simulink model "RMU22"  (R2025b)
settings: Solver=VariableStepAuto  StartTime=0.0  StopTime=12  RelTol=1e-3
libraries: spsThreePhaseBreakerLib x11, spsThreePhaseParallelRLCLoadLib x6, spsThreePhasePISectionLineLib x6, spsThreePhaseFaultLib x3, spsThreePhaseVIMeasurementLib x3, spsThreePhaseSourceLib x2, spsThreePhaseTransformerTwoWindingsLib x2, sps_lib x1
settings Model: Creator=sheya  LastModifiedBy=josna_mz

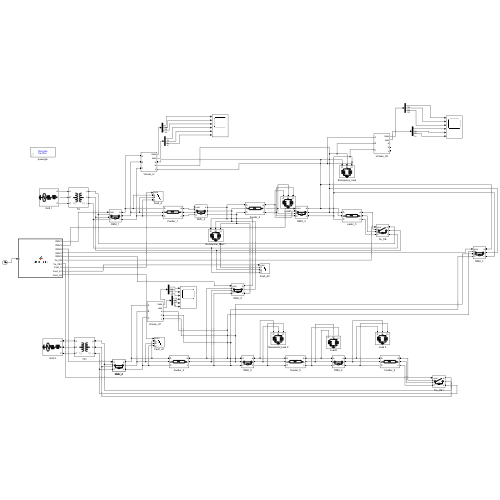
[thumbnail: Simulink's stored preview of the top-level diagram]
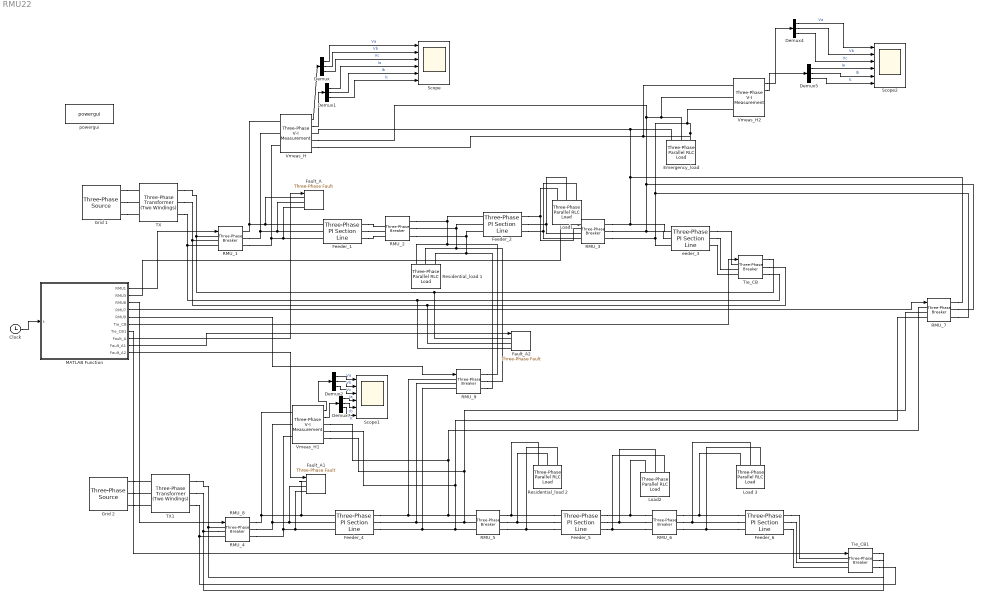
== system RMU22 ==
  Clock : Clock
  Demux{,1..5} (6 alike) : Demux  Outputs=3
  Emergency_load : spsThreePhaseParallelRLCLoadLib/Three-Phase Parallel RLC Load  LConnTagsString=A|B|C  Configuration=Y (grounded)  NominalVoltage=11000  Vabc=[1e3 1e3 1e3]  Vabcp=[1e3 1e3 1e3]  NominalFrequency=60  UnbalancedPower=off  ActivePower=5e5  InductivePower=1.64e5  CapacitivePower=0  Pabc=[10e3 9e3 11e3]  QLabc=[100 90 110]  QCabc=[100 90 110]  Pabcp=[10e3 9e3 11e3]  QLabcp=[100 90 110]  QCabcp=[100 90 110]  Measurements=None  LoadType=constant Z
  Fault_A : spsThreePhaseFaultLib/Three-Phase Fault  InitialStates=0  FaultA=on  FaultB=on  FaultC=on  GroundFault=on  SwitchTimes="[0.2  0.5]"  External=on  SwitchStatus=NaN  FaultResistance=0.001  GroundResistance=0.01  SnubberResistance=1e6  SnubberCapacitance=inf  Measurements=None
  Fault_A1 : spsThreePhaseFaultLib/Three-Phase Fault  InitialStates=0  FaultA=on  FaultB=on  FaultC=on  GroundFault=on  SwitchTimes="[0.2  0.5]"  External=on  SwitchStatus=NaN  FaultResistance=0.001  GroundResistance=0.01  SnubberResistance=1e6  SnubberCapacitance=inf  Measurements=None
  Fault_A2 : spsThreePhaseFaultLib/Three-Phase Fault  InitialStates=0  FaultA=on  FaultB=on  FaultC=on  GroundFault=on  SwitchTimes="[0.2  0.5]"  External=on  SwitchStatus=NaN  FaultResistance=0.001  GroundResistance=0.01  SnubberResistance=1e6  SnubberCapacitance=inf  Measurements=None
  Feeder_{1..2,4..6} (5 alike) : spsThreePhasePISectionLineLib/Three-Phase PI Section Line  LConnTagsString=a|b|c  RConnTagsString=A|B|C  Length=100  Frequency=60  Resistances=[ 0.01273 0.3864]  Inductances="[ 0.9337e-3  4.1264e-3]"  Capacitances=[12.74e-9 7.751e-9]
  Grid 1 : spsThreePhaseSourceLib/Three-Phase Source  InternalConnection=Yg  VoltagePhases=off  Voltage=11000  PhaseAngle=0  Voltage_phases=[25e3 25e3 25e3]/sqrt(3)  PhaseAngles_phases=[0 -120 +120]  Frequency=50  NonIdealSource=on  SpecifyImpedance=off  Resistance=0.8929  Inductance=16.58e-3  ShortCircuitLevel=100e6  BaseVoltage=25e3  XRratio=7  BusType=swing  Pref=10e3  Qref=0  Prefabc=[10e3, 10e3, 10e3]  Qrefabc=[0, 0, 0]  Qmin=-inf  Qmax=inf
  Grid 2 : spsThreePhaseSourceLib/Three-Phase Source  InternalConnection=Yg  VoltagePhases=off  Voltage=11000  PhaseAngle=0  Voltage_phases=[25e3 25e3 25e3]/sqrt(3)  PhaseAngles_phases=[0 -120 +120]  Frequency=50  NonIdealSource=on  SpecifyImpedance=off  Resistance=0.8929  Inductance=16.58e-3  ShortCircuitLevel=100e6  BaseVoltage=25e3  XRratio=7  BusType=swing  Pref=10e3  Qref=0  Prefabc=[10e3, 10e3, 10e3]  Qrefabc=[0, 0, 0]  Qmin=-inf  Qmax=inf
  Load 3 : spsThreePhaseParallelRLCLoadLib/Three-Phase Parallel RLC Load  LConnTagsString=A|B|C  Configuration=Y (grounded)  NominalVoltage=11000  Vabc=[1e3 1e3 1e3]  Vabcp=[1e3 1e3 1e3]  NominalFrequency=60  UnbalancedPower=off  ActivePower=7e5  InductivePower=3.77e5  CapacitivePower=0  Pabc=[10e3 9e3 11e3]  QLabc=[100 90 110]  QCabc=[100 90 110]  Pabcp=[10e3 9e3 11e3]  QLabcp=[100 90 110]  QCabcp=[100 90 110]  Measurements=None  LoadType=constant Z
  Load1 : spsThreePhaseParallelRLCLoadLib/Three-Phase Parallel RLC Load  LConnTagsString=A|B|C  Configuration=Y (grounded)  NominalVoltage=11000  Vabc=[1e3 1e3 1e3]  Vabcp=[1e3 1e3 1e3]  NominalFrequency=60  UnbalancedPower=off  ActivePower=6e5  InductivePower=3.71e5  CapacitivePower=0  Pabc=[10e3 9e3 11e3]  QLabc=[100 90 110]  QCabc=[100 90 110]  Pabcp=[10e3 9e3 11e3]  QLabcp=[100 90 110]  QCabcp=[100 90 110]  Measurements=None  LoadType=constant Z
  Load2 : spsThreePhaseParallelRLCLoadLib/Three-Phase Parallel RLC Load  LConnTagsString=A|B|C  Configuration=Y (grounded)  NominalVoltage=11000  Vabc=[1e3 1e3 1e3]  Vabcp=[1e3 1e3 1e3]  NominalFrequency=60  UnbalancedPower=off  ActivePower=5e5  InductivePower=2.42e5  CapacitivePower=0  Pabc=[10e3 9e3 11e3]  QLabc=[100 90 110]  QCabc=[100 90 110]  Pabcp=[10e3 9e3 11e3]  QLabcp=[100 90 110]  QCabcp=[100 90 110]  Measurements=None  LoadType=constant Z
  MATLAB Function : MATLAB Function  TreatAsAtomicUnit=on
  RMU_{1..4,7,9} (6 alike) : spsThreePhaseBreakerLib/Three-Phase Breaker  InitialState=closed  SwitchA=on  SwitchB=on  SwitchC=on  SwitchTimes="[1/60  5/60]"  External=on  BreakerResistance=0.01  SnubberResistance=1e6  SnubberCapacitance=inf  Measurements=None
  RMU_5 : spsThreePhaseBreakerLib/Three-Phase Breaker  InitialState=closed  SwitchA=on  SwitchB=on  SwitchC=on  SwitchTimes="[1/60  5/60]"  External=off  BreakerResistance=0.01  SnubberResistance=1e6  SnubberCapacitance=inf  Measurements=None
  RMU_6 : spsThreePhaseBreakerLib/Three-Phase Breaker  InitialState=closed  SwitchA=on  SwitchB=on  SwitchC=on  SwitchTimes="[1/60  5/60]"  External=off  BreakerResistance=0.01  SnubberResistance=1e6  SnubberCapacitance=inf  Measurements=None
  RMU_8 : spsThreePhaseBreakerLib/Three-Phase Breaker  InitialState=closed  SwitchA=on  SwitchB=on  SwitchC=on  SwitchTimes="[1/60  5/60]"  External=off  BreakerResistance=0.01  SnubberResistance=1e6  SnubberCapacitance=inf  Measurements=None
  Residential_load 1 : spsThreePhaseParallelRLCLoadLib/Three-Phase Parallel RLC Load  LConnTagsString=A|B|C  Configuration=Y (grounded)  NominalVoltage=11000  Vabc=[1e3 1e3 1e3]  Vabcp=[1e3 1e3 1e3]  NominalFrequency=60  UnbalancedPower=off  ActivePower=9e5  InductivePower=4.36e5  CapacitivePower=0  Pabc=[10e3 9e3 11e3]  QLabc=[100 90 110]  QCabc=[100 90 110]  Pabcp=[10e3 9e3 11e3]  QLabcp=[100 90 110]  QCabcp=[100 90 110]  Measurements=None  LoadType=constant Z
  Residential_load 2 : spsThreePhaseParallelRLCLoadLib/Three-Phase Parallel RLC Load  LConnTagsString=A|B|C  Configuration=Y (grounded)  NominalVoltage=11000  Vabc=[1e3 1e3 1e3]  Vabcp=[1e3 1e3 1e3]  NominalFrequency=60  UnbalancedPower=off  ActivePower=8e5  InductivePower=3.87e5  CapacitivePower=0  Pabc=[10e3 9e3 11e3]  QLabc=[100 90 110]  QCabc=[100 90 110]  Pabcp=[10e3 9e3 11e3]  QLabcp=[100 90 110]  QCabcp=[100 90 110]  Measurements=None  LoadType=constant Z
  Scope : Scope  NumInputPorts=6
      settings: ActiveDisplayYMinimum=-1  ActiveDisplayYMaximum=1  YLabel=Voltage (Volts)
  Scope1 : Scope  NumInputPorts=6
      settings: ActiveDisplayYMinimum=-6112.8015624898089  ActiveDisplayYMaximum=6194.6590194442269  YLabel=Voltage (Volts)
  Scope2 : Scope  NumInputPorts=6
      settings: ActiveDisplayYMinimum=-1  ActiveDisplayYMaximum=1  YLabel=Voltage (Volts)  DataLoggingVariableName=ScopeData2
  TX : spsThreePhaseTransformerTwoWindingsLib/Three-Phase Transformer (Two Windings)  Winding1Connection=Yg  Winding2Connection=Yg  CoreType=Three single-phase transformers  SetSaturation=off  Hysteresis=off  DataFile='hysteresis'  SetInitialFlux=off  Measurements=None  UNITS=pu  NominalPower=[ 250e6 , 60 ]  Winding1=[ 735e3 , 0.002 , 0.08 ]  Winding2=[ 315e3 , 0.002 , 0.08 ]  Rm=500  Lm=500  L0=0.5  Saturation=[ 0,0 ; 0.0024,1.2 ; 1.0,1.52 ]  InitialFluxes=[ 0.8 , -0.8 , 0.7 ]  BreakLoop=off  DiscreteSolver=Trapezoidal iterative  DataType=off  TransfoNumber=1
  TX1 : spsThreePhaseTransformerTwoWindingsLib/Three-Phase Transformer (Two Windings)  Winding1Connection=Yg  Winding2Connection=Yg  CoreType=Three single-phase transformers  SetSaturation=off  Hysteresis=off  DataFile='hysteresis'  SetInitialFlux=off  Measurements=None  UNITS=pu  NominalPower=[ 250e6 , 60 ]  Winding1=[ 735e3 , 0.002 , 0.08 ]  Winding2=[ 315e3 , 0.002 , 0.08 ]  Rm=500  Lm=500  L0=0.5  Saturation=[ 0,0 ; 0.0024,1.2 ; 1.0,1.52 ]  InitialFluxes=[ 0.8 , -0.8 , 0.7 ]  BreakLoop=off  DiscreteSolver=Trapezoidal iterative  DataType=off  TransfoNumber=1
  Tie_CB : spsThreePhaseBreakerLib/Three-Phase Breaker  InitialState=open  SwitchA=on  SwitchB=on  SwitchC=on  SwitchTimes="[1/60  5/60]"  External=on  BreakerResistance=0.01  SnubberResistance=1e6  SnubberCapacitance=inf  Measurements=None
  Tie_CB1 : spsThreePhaseBreakerLib/Three-Phase Breaker  InitialState=open  SwitchA=on  SwitchB=on  SwitchC=on  SwitchTimes="[1/60  5/60]"  External=on  BreakerResistance=0.01  SnubberResistance=1e6  SnubberCapacitance=inf  Measurements=None
  Vmeas_H : spsThreePhaseVIMeasurementLib/Three-Phase V-I Measurement  VoltageMeasurement=phase-to-ground  SetLabelV=off  LabelV=Vabc  Vpu=off  VpuLL=off  CurrentMeasurement=yes  SetLabelI=off  LabelI=Iabc  Ipu=off  Pbase=100e6  Vbase=500e3  OutputType=Complex  PhasorSimulation=off  PSBequivalent=0
  Vmeas_H1 : spsThreePhaseVIMeasurementLib/Three-Phase V-I Measurement  VoltageMeasurement=phase-to-ground  SetLabelV=off  LabelV=Vabc  Vpu=off  VpuLL=off  CurrentMeasurement=yes  SetLabelI=off  LabelI=Iabc  Ipu=off  Pbase=100e6  Vbase=500e3  OutputType=Complex  PhasorSimulation=off  PSBequivalent=0
  Vmeas_H2 : spsThreePhaseVIMeasurementLib/Three-Phase V-I Measurement  VoltageMeasurement=phase-to-ground  SetLabelV=off  LabelV=Vabc  Vpu=off  VpuLL=off  CurrentMeasurement=yes  SetLabelI=off  LabelI=Iabc  Ipu=off  Pbase=100e6  Vbase=500e3  OutputType=Complex  PhasorSimulation=off  PSBequivalent=0
  eeder_3 : spsThreePhasePISectionLineLib/Three-Phase PI Section Line  LConnTagsString=a|b|c  RConnTagsString=A|B|C  Length=100  Frequency=60  Resistances=[ 0.01273 0.3864]  Inductances="[ 0.9337e-3  4.1264e-3]"  Capacitances=[12.74e-9 7.751e-9]
  powergui : sps_lib/powergui  Priority=1  SimulationMode=Discrete  SampleTime=50e-6  frequency=60  Iterations=50  frequencyindice=0  Pbase=100e6  ErrMax=1e-4  UnitsV=kV  UnitsW=MW  buscounter=0  FunctionMessages=off  echomessages=off  EnableUseOfTLC=off  CurrentSourceSwitches=off  DisableSnubberDevices=off  DisableRonSwitches=off  DisableVfSwitches=off  DisplayEquations=off  AutomaticDiscreteSolvers=off  SolverType=Tustin/Backward Euler (TBE)  Interpol=off  ExternalGateDelay=off  methode=off  Ts=100  x0status=blocks  SPID=on  SwTol=0  HookPort=off  NonlinearTolerance=1e-4  nMaxIteration=100  ContinueOnMaxIteration=off  RestoreLinks=warning  ResistiveCurrentMeasurement=off  Frange=[0:2:500]  Ylog=off  Xlog=on  ShowGrid=off  save=off  variable=ZData  structure=0  ZoomFFT=off  StartTime=0.0  cycles=1  DisplayStyle=1  fundamental=60  FreqAxis=off  MaxFrequency=1000  frequencyindicesteady=1  RmsSteady=1  display=off
  wires:
  Vmeas_H/1 -> Demux/1
  Demux/1 -> Scope/1  "Va"
  Demux/2 -> Scope/2  "Vb"
  Demux/3 -> Scope/3  "Vc"
  Demux1/1 -> Scope/4  "Ia"
  Demux1/2 -> Scope/5  "Ib"
  Demux1/3 -> Scope/6  "Ic"
  Vmeas_H/2 -> Demux1/1
  Demux3/2 -> Scope1/5  "Ib"
  Demux3/3 -> Scope1/6  "Ic"
  Demux2/3 -> Scope1/3  "Vc"
  Demux2/2 -> Scope1/2  "Vb"
  Vmeas_H1/2 -> Demux3/1
  Vmeas_H1/1 -> Demux2/1
  Demux2/1 -> Scope1/1  "Va"
  Demux3/1 -> Scope1/4  "Ia"
  MATLAB Function/1(RMU1) -> RMU_1/1
  MATLAB Function/6(Tie_CB) -> Tie_CB/1
  MATLAB Function/4(RMU7) -> RMU_7/1
  Clock/1 -> MATLAB Function/1(t)
  MATLAB Function/2(RMU3) -> RMU_3/1
  MATLAB Function/5(RMU9) -> RMU_9/1
  MATLAB Function/7(Tie_CB1) -> Tie_CB1/1
  MATLAB Function/8(Fault_A) -> Fault_A/1
  MATLAB Function/9(Fault_A1) -> Fault_A2/1
  MATLAB Function/10(Fault_A2) -> Fault_A1/1
  MATLAB Function/3(RMU8) -> RMU_4/1
  Vmeas_H2/1 -> Demux4/1
  Vmeas_H2/2 -> Demux5/1
  Demux4/1 -> Scope2/1  "Va"
  Demux4/2 -> Scope2/2  "Vb"
  Demux4/3 -> Scope2/3  "Vc"
  Demux5/1 -> Scope2/4  "Ia"
  Demux5/2 -> Scope2/5  "Ib"
  Demux5/3 -> Scope2/6  "Ic"
  connections:
  Grid 1/RConn1 -- TX/LConn1
  TX/RConn1 -- Fault_A2/LConn1 -- Tie_CB/RConn1 -- RMU_1/LConn1
  RMU_1/RConn1 -- Vmeas_H/LConn1 -- Fault_A/LConn1 -- Feeder_1/LConn1
  Feeder_1/RConn1 -- RMU_2/LConn1
  RMU_2/RConn1 -- RMU_9/RConn1 -- Residential_load 1/LConn1 -- Feeder_2/LConn1
  Feeder_2/RConn1 -- RMU_3/LConn1 -- Load1/LConn1
  RMU_3/RConn1 -- Emergency_load/LConn1 -- Vmeas_H/RConn1 -- RMU_7/RConn1 -- eeder_3/LConn1
  eeder_3/RConn1 -- Tie_CB/LConn1
  eeder_3/RConn2 -- Tie_CB/LConn2
  eeder_3/RConn3 -- Tie_CB/LConn3
  TX/RConn2 -- Tie_CB/RConn2 -- Fault_A2/LConn2 -- RMU_1/LConn2
  TX/RConn3 -- Fault_A2/LConn3 -- Tie_CB/RConn3 -- RMU_1/LConn3
  Grid 1/RConn2 -- TX/LConn2
  Grid 1/RConn3 -- TX/LConn3
  RMU_2/RConn2 -- RMU_9/RConn2 -- Residential_load 1/LConn2 -- Feeder_2/LConn2
  RMU_2/RConn3 -- RMU_9/RConn3 -- Residential_load 1/LConn3 -- Feeder_2/LConn3
  Feeder_2/RConn2 -- RMU_3/LConn2 -- Load1/LConn2
  Feeder_2/RConn3 -- RMU_3/LConn3 -- Load1/LConn3
  RMU_3/RConn2 -- Vmeas_H2/LConn2 -- Emergency_load/LConn2 -- Vmeas_H/RConn2 -- RMU_7/RConn2 -- eeder_3/LConn2
  RMU_3/RConn3 -- Vmeas_H2/LConn3 -- Vmeas_H2/LConn1 -- Vmeas_H/RConn3 -- Emergency_load/LConn3 -- RMU_7/RConn3 -- eeder_3/LConn3
  RMU_1/RConn2 -- Feeder_1/LConn2 -- Fault_A/LConn2 -- Vmeas_H/LConn2
  RMU_1/RConn3 -- Vmeas_H/LConn3 -- Feeder_1/LConn3 -- Fault_A/LConn3
  Feeder_1/RConn2 -- RMU_2/LConn2
  Feeder_1/RConn3 -- RMU_2/LConn3
  RMU_6/LConn2 -- Feeder_5/RConn2 -- Load2/LConn2
  Feeder_5/LConn1 -- RMU_5/RConn1 -- Residential_load 2/LConn1
  RMU_4/RConn1 -- Vmeas_H1/LConn1 -- Fault_A1/LConn1 -- Feeder_4/LConn1
  RMU_6/LConn1 -- Feeder_5/RConn1 -- Load2/LConn1
  Feeder_6/LConn3 -- RMU_6/RConn3 -- Load 3/LConn3
  Fault_A1/LConn3 -- Feeder_4/LConn3 -- RMU_4/RConn3 -- Vmeas_H1/LConn3
  Vmeas_H1/LConn2 -- RMU_4/RConn2 -- Feeder_4/LConn2 -- Fault_A1/LConn2
  Feeder_6/LConn2 -- RMU_6/RConn2 -- Load 3/LConn2
  Feeder_6/LConn1 -- RMU_6/RConn1 -- Load 3/LConn1
  TX1/RConn3 -- Tie_CB1/RConn3 -- RMU_4/LConn3
  Feeder_5/LConn3 -- RMU_5/RConn3 -- Residential_load 2/LConn3
  RMU_6/LConn3 -- Feeder_5/RConn3 -- Load2/LConn3
  RMU_4/LConn2 -- TX1/RConn2 -- Tie_CB1/RConn2
  Feeder_5/LConn2 -- RMU_5/RConn2 -- Residential_load 2/LConn2
  TX1/RConn1 -- Tie_CB1/RConn1 -- RMU_4/LConn1
  Feeder_6/RConn2 -- Tie_CB1/LConn2
  Feeder_6/RConn1 -- Tie_CB1/LConn1
  Feeder_6/RConn3 -- Tie_CB1/LConn3
  Grid 2/RConn1 -- TX1/LConn1
  Feeder_4/RConn1 -- RMU_9/LConn1 -- RMU_7/LConn1 -- Vmeas_H1/RConn1 -- RMU_5/LConn1
  Feeder_4/RConn2 -- RMU_9/LConn2 -- RMU_7/LConn2 -- Vmeas_H1/RConn3 -- RMU_5/LConn2
  Grid 2/RConn3 -- TX1/LConn3
  Feeder_4/RConn3 -- RMU_9/LConn3 -- RMU_7/LConn3 -- Vmeas_H1/RConn2 -- RMU_5/LConn3
  Grid 2/RConn2 -- TX1/LConn2

== matlab function RMU22/MATLAB Function ==
  data: RMU1 output; RMU3 output; RMU8 output; RMU7 output; RMU9 output; Tie_CB output; Tie_CB1 output; Fault_A output; t input; Fault_A1 output; Fault_A2 output
function [RMU1, RMU3, RMU8, RMU7, RMU9, Tie_CB, Tie_CB1, Fault_A, Fault_A1, Fault_A2] = control_logic(t)

% INITIAL STATE (Normal condition)
RMU1 = 1;     
RMU3 = 1;
RMU8 = 1;
RMU7 = 1;
RMU9 = 0;     

Tie_CB = 0;   
Tie_CB1 = 0;

Fault_A = 0;
Fault_A1 = 0;
Fault_A2 = 0;

%% ----------- TIME BASED FAULT SCENARIOS (5 sec each) -----------

% 1. Fault A (Short circuit / Line fault in Grid 1)
if (t >= 3 && t < 6)
    Fault_A = 1;

    RMU1 = 0;        
    Tie_CB = 1;      
end

% 2. Transient / Overvoltage (Oscillation case)
if (t >= 7 && t < 9)
    Fault_A = 1;

    % Oscillation effect
    if mod(floor(t*10),2) == 0
        RMU1 = 0;
        Tie_CB = 1;
    else
        RMU1 = 1;
        Tie_CB = 0;
    end
end

% 3. Severe Fault (Blackout condition - Grid 1 failure)
if (t >= 11 && t < 16)
    Fault_A = 1;
    Fault_A2 = 1;

    RMU1 = 0;
    Tie_CB = 0;

    % Supply only from Grid 2
    RMU7 = 1;
end

% 4. Overload in Grid 1
if (t >= 16 && t < 21)
    RMU9 = 1;   
end

% 5. Grid 2 Fault (Fault_A1)
if (t >= 21 && t < 26)
    Fault_A1 = 1;

    RMU8 = 0;       
    Tie_CB1 = 1;    
end

% 6. System Restoration
if (t >= 26)
    RMU1 = 1;
    RMU3 = 1;
    RMU8 = 1;
    RMU7 = 1;
    RMU9 = 0;

    Tie_CB = 0;
    Tie_CB1 = 0;

    Fault_A = 0;
    Fault_A1 = 0;
    Fault_A2 = 0;
end

end
